simulink model "Lead_Lag_Controller"  (R2020b)
settings: Solver=VariableStepAuto  StartTime=0.0  StopTime=100  RelTol=1e-3
values from neighbouring files (symbols this model uses):
  s = tf('s')    [Test_longitudinal.m]
libraries: slctrlblks x3, simulink x3
settings Model: Creator=99003747  LastModifiedBy=99003747

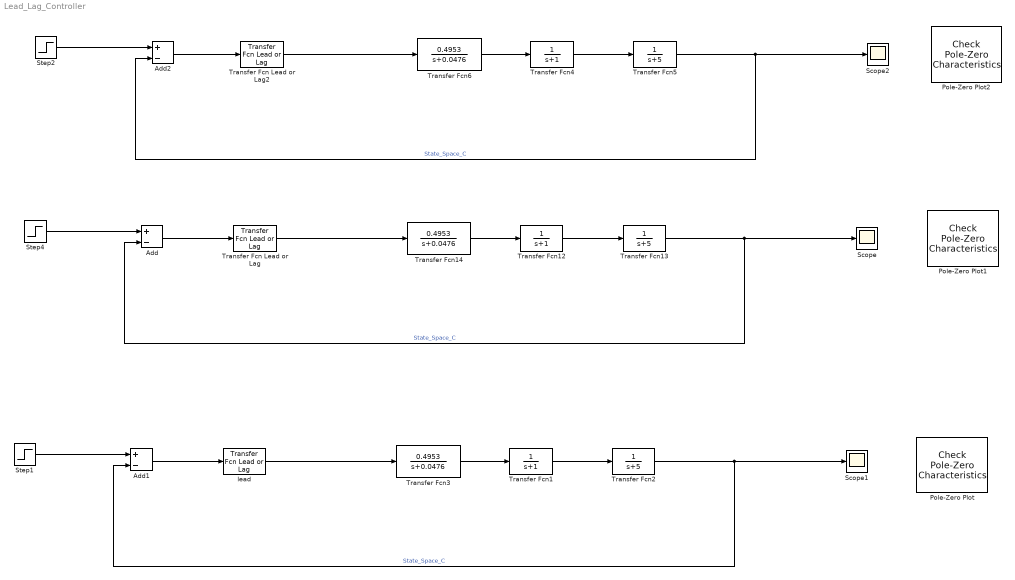
== system Lead_Lag_Controller ==
  Add : Sum  Inputs=+-
  Add1 : Sum  Inputs=+-
  Add2 : Sum  Inputs=+-
  Pole-Zero Plot : slctrlblks/Model Verification/Check Pole-Zero Characteristics  InstantiateOnLoad=on  SaveOperatingPoints=off  LinearizationIOs={'/Step1', 1, 'in', 'off', '';'/Transfer Fcn2', 1, 'out', 'off', ''}  LinearizeAt=SnapshotTimes  SnapshotTimes=[0]  TriggerType=rising  SampleTime=auto  RateConversionMethod=zoh  PreWarpFreq=10  UseExactDelayModel=off  UseFullBlockNameLabels=off  UseBusSignalLabels=off  enabled=on  stopWhenAssertionFail=off  export=off  ViewDlgPos=[1 41 1920 963]  LaunchViewOnOpen=on  OpenViewOnLoad=off  FrequencyUnits=rad/s  MagnitudeUnits=dB  PhaseUnits=deg  TimeUnits=seconds  EnableSettlingTime=off  SettlingTime=[]  EnablePercentOvershoot=off  PercentOvershoot=[]  EnableDampingRatio=off  DampingRatio=[]  EnableNaturalFrequency=off  NaturalFrequencyBound=>=  NaturalFrequency=[]
      settings: SourceProductBaseCode=SD  SaveToWorkspace=off  SaveName=sys
  Pole-Zero Plot1 : slctrlblks/Model Verification/Check Pole-Zero Characteristics  InstantiateOnLoad=on  SaveOperatingPoints=off  LinearizationIOs={'/Transfer Fcn13', 1, 'out', 'off', '';'/Step4', 1, 'in', 'off', ''}  LinearizeAt=SnapshotTimes  SnapshotTimes=[0]  TriggerType=rising  SampleTime=auto  RateConversionMethod=zoh  PreWarpFreq=10  UseExactDelayModel=off  UseFullBlockNameLabels=off  UseBusSignalLabels=off  enabled=on  stopWhenAssertionFail=off  export=off  ViewDlgPos=[1 41 1920 963]  LaunchViewOnOpen=on  OpenViewOnLoad=off  FrequencyUnits=rad/s  MagnitudeUnits=dB  PhaseUnits=deg  TimeUnits=seconds  EnableSettlingTime=off  SettlingTime=[]  EnablePercentOvershoot=off  PercentOvershoot=[]  EnableDampingRatio=off  DampingRatio=[]  EnableNaturalFrequency=off  NaturalFrequencyBound=>=  NaturalFrequency=[]
      settings: SourceProductBaseCode=SD  SaveToWorkspace=off  SaveName=sys
  Pole-Zero Plot2 : slctrlblks/Model Verification/Check Pole-Zero Characteristics  InstantiateOnLoad=on  SaveOperatingPoints=off  LinearizationIOs={'/Transfer Fcn5', 1, 'out', 'off', '';'/Step2', 1, 'in', 'off', ''}  LinearizeAt=SnapshotTimes  SnapshotTimes=[0]  TriggerType=rising  SampleTime=auto  RateConversionMethod=zoh  PreWarpFreq=10  UseExactDelayModel=off  UseFullBlockNameLabels=off  UseBusSignalLabels=off  enabled=on  stopWhenAssertionFail=off  export=off  ViewDlgPos=[1 41 1920 963]  LaunchViewOnOpen=on  OpenViewOnLoad=off  FrequencyUnits=rad/s  MagnitudeUnits=dB  PhaseUnits=deg  TimeUnits=seconds  EnableSettlingTime=off  SettlingTime=[]  EnablePercentOvershoot=off  PercentOvershoot=[]  EnableDampingRatio=off  DampingRatio=[]  EnableNaturalFrequency=off  NaturalFrequencyBound=>=  NaturalFrequency=[]
      settings: SourceProductBaseCode=SD  SaveToWorkspace=off  SaveName=sys
  Scope : Scope
  Scope1 : Scope
  Scope2 : Scope
  Step1 : Step  After=30  SampleTime=0
  Step2 : Step  After=30  SampleTime=0
  Step4 : Step  After=30  SampleTime=0
  Transfer Fcn Lead or Lag : simulink/Discrete/Transfer Fcn Lead or Lag  PoleZ=(0.95)  ZeroZ=0  ICPrevOutput=0.0  ICPrevInput=0.0  DoSatur=off
      settings: SourceProductBaseCode=SL
  Transfer Fcn Lead or Lag2 : simulink/Discrete/Transfer Fcn Lead or Lag  PoleZ=0.95  ZeroZ=0.75  ICPrevOutput=0.0  ICPrevInput=0.0  DoSatur=off
      settings: SourceProductBaseCode=SL
  Transfer Fcn1 : TransferFcn  Denominator=[1 1]
  Transfer Fcn12 : TransferFcn  Denominator=[1 1]
  Transfer Fcn13 : TransferFcn  Denominator=[1 5]
  Transfer Fcn14 : TransferFcn  Numerator=[0.4953]  Denominator=[1 0.0476]
  Transfer Fcn2 : TransferFcn  Denominator=[1 5]
  Transfer Fcn3 : TransferFcn  Numerator=[0.4953]  Denominator=[1 0.0476]
  Transfer Fcn4 : TransferFcn  Denominator=[1 1]
  Transfer Fcn5 : TransferFcn  Denominator=[1 5]
  Transfer Fcn6 : TransferFcn  Numerator=[0.4953]  Denominator=[1 0.0476]
  lead : simulink/Discrete/Transfer Fcn Lead or Lag  PoleZ=0  ZeroZ=0.75  ICPrevOutput=0.0  ICPrevInput=0.0  DoSatur=off
      settings: SourceProductBaseCode=SL
  wires:
  Add/1 -> Transfer Fcn Lead or Lag/1
  Step4/1 -> Add/1
  Transfer Fcn Lead or Lag/1 -> Transfer Fcn14/1
  Transfer Fcn14/1 -> Transfer Fcn12/1
  Transfer Fcn13/1 -> Scope/1, Add/2  "State_Space_C"
  Transfer Fcn12/1 -> Transfer Fcn13/1
  Transfer Fcn3/1 -> Transfer Fcn1/1
  Add1/1 -> lead/1
  Step1/1 -> Add1/1
  Transfer Fcn2/1 -> Scope1/1, Add1/2  "State_Space_C"
  lead/1 -> Transfer Fcn3/1
  Transfer Fcn1/1 -> Transfer Fcn2/1
  Transfer Fcn6/1 -> Transfer Fcn4/1
  Step2/1 -> Add2/1
  Transfer Fcn5/1 -> Scope2/1, Add2/2  "State_Space_C"
  Transfer Fcn Lead or Lag2/1 -> Transfer Fcn6/1
  Transfer Fcn4/1 -> Transfer Fcn5/1
  Add2/1 -> Transfer Fcn Lead or Lag2/1
